simulink model "on_line_dyskretny_zmienny_18"  (R2018b)
settings: Solver=VariableStepAuto  StartTime=0.0  StopTime=20  RelTol=1e-3
model workspace (MAT data in the model file):
  denom = Simulink.Parameter
  denom.Value = [1 0.3 0.4]
  denom.DataType = 'auto'
  denom.Dimensions = [1 3]
libraries: ctrlSharedLib x1
settings Model: Creator=Dominik  LastModifiedBy=user
settings SFSimCC: SimUseLocalCustomCode=off
settings RTWCC: RTWUseLocalCustomCode=off

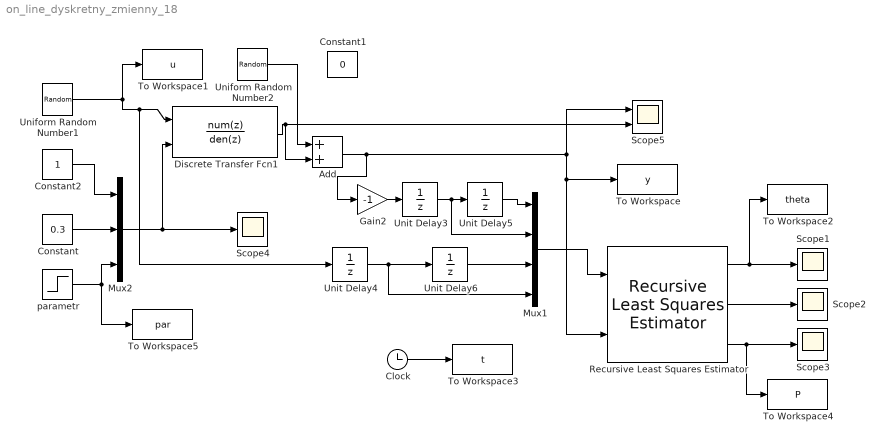
== system on_line_dyskretny_zmienny_18 ==
  Add : Sum
  Clock : Clock
  Constant : Constant  Value=0.3
  Constant1 : Constant  Value=0
  Constant2 : Constant
  Discrete Transfer Fcn1 : DiscreteTransferFcn  Numerator=[0.1 0.2]  DenominatorSource=Input port  Denominator=[1 0.3 0.4]  a0EqualsOne=on
      settings: InputPortMap=u0,p3
  Gain2 : Gain  Gain=-1
  Mux1 : Mux
  Mux2 : Mux  Inputs=3
  Recursive Least Squares Estimator : ctrlSharedLib/Recursive Least Squares Estimator  InitialEstimateSource=None  InitialParameterData=4  P0=10000  InitialRegressors=0  InitialOutputs=0  History=Infinite  WindowLength=200  EstimationMethod=Forgetting Factor  AdaptationParameter=0.96  HasTimeVaryingAdaptationParameter=off  NormalizationBias=eps  OutputError=on  OutputP=on  AddEnablePort=off  InputProcessing=Sample-based  Ts=-1
      settings: SourceProductName=Control System Toolbox  SourceProductBaseCode=CT
  Scope{1..4} (4 alike) : Scope
  Scope5 : Scope  NumInputPorts=2
  To Workspace : ToWorkspace  VariableName=y  SampleTime=-1
  To Workspace1 : ToWorkspace  VariableName=u  SampleTime=-1
  To Workspace2 : ToWorkspace  VariableName=theta  SampleTime=-1
  To Workspace3 : ToWorkspace  VariableName=t  SampleTime=-1
  To Workspace4 : ToWorkspace  VariableName=P  SampleTime=-1
  To Workspace5 : ToWorkspace  VariableName=par  SampleTime=-1
  Uniform Random Number1 : UniformRandomNumber  SampleTime=0.1
  Uniform Random Number2 : UniformRandomNumber  Minimum=-0.01  Maximum=0.01  Seed=3214  SampleTime=0.1
  Unit Delay{3..6} (4 alike) : UnitDelay  SampleTime=-1
  parametr : Step  Time=10  Before=0.4  After=0.25  SampleTime=0
  wires:
  Recursive Least Squares Estimator/1 -> Scope1/1, To Workspace2/1
  Clock/1 -> To Workspace3/1
  Recursive Least Squares Estimator/3 -> To Workspace4/1, Scope3/1
  parametr/1 -> To Workspace5/1, Mux2/3
  Unit Delay3/1 -> Mux1/2, Unit Delay5/1
  Gain2/1 -> Unit Delay3/1
  Unit Delay5/1 -> Mux1/1
  Mux1/1 -> Recursive Least Squares Estimator/1
  Unit Delay4/1 -> Mux1/4, Unit Delay6/1
  Unit Delay6/1 -> Mux1/3
  Constant/1 -> Mux2/2
  Uniform Random Number1/1 -> Discrete Transfer Fcn1/1, Unit Delay4/1, To Workspace1/1
  Mux2/1 -> Discrete Transfer Fcn1/2, Scope4/1
  Uniform Random Number2/1 -> Add/1
  Discrete Transfer Fcn1/1 -> Add/2, Scope5/2
  Add/1 -> Scope5/1, Recursive Least Squares Estimator/2, To Workspace/1, Gain2/1
  Constant2/1 -> Mux2/1
  Recursive Least Squares Estimator/2 -> Scope2/1
